simulink model "LoFT_Example3"  (R2024b)
settings: Solver=ode4  StartTime=0.0  StopTime=300  FixedStep=simu.dt  RelTol=1e-3
undefined symbols (not defined in the file): body, circtime, Communication, D1, Delta, irkb, line, LoFT, p0, Pn, s, simu, trip_time, Turbwind, waves, wind
libraries: simulink x350, spsThreePhaseVIMeasurementLib x41, spsThreePhasePISectionLineLib x34, spsThreePhaseParallelRLCLoadLib x21, spsThreePhaseTransformerTwoWindingsLib x14, spsLoadFlowBusLib x10, spsThreePhaseDynamicLoadLib x9, spsSynchronousMachinepuStandardLib x7, spsExcitationSystemLib x7, spsSteamTurbineandGovernorLib x7, spsGenericPowerSystemStabilizerLib x7, spsMultiBandPowerSystemStabilizerLib x7
(part 40 of 49)

== system LoFT_Example3/FOWT System/Subsystem11/FOWT6/Aerodynamics and Local Control Systems/Local Control Systems/Subsystem1 ==
  RotSpeed : Inport
  WindSpeed : Inport  Port=2
  3 : Inport  Port=3
  Nacelle Speed : Inport  Port=4
  1-D Lookup Table : Lookup_n-D  NumberOfTableDimensions=1  BreakpointsForDimension1=Controller.R.PS_WindSpeeds  Table=Controller.R.PS_BldPitchMin  InternalRulePriority=Speed  RndMeth=Simplest
  Compare To Constant : simulink/Logic and Bit Operations/Compare To Constant  relop=<=  const=0  OutDataTypeStr=boolean
  Constant : Constant  Value=7.55*pi/30
  Constant1 : Constant  Value=90*pi/180
  Delay : Delay  DelayLength=1  InitialCondition=0
  Divide3 : Product  Inputs=**
  Gain : Gain  Gain=Controller.KV *0.5
  Gain Scheduling : Subsystem
  Gain1 : Gain
  Rate Limiter : RateLimiter  RisingSlewLimit=2*pi/180  FallingSlewLimit=-2 * pi/180  SampleTimeMode=inherited
  Saturation : Saturate  UpperLimit=7.55*pi/30  LowerLimit=5*pi/30
  Saturation Dynamic : simulink/Discontinuities/Saturation Dynamic  OutMin=[]  OutMax=[]  OutDataTypeStr=Inherit: Same as second input  OutDataType=fixdt(1, 16)  OutScaling=2^-10  DoSatur=off
  Scope2 : Scope
  Sum1 : Sum  Inputs=|++
  Sum3 : Sum  Inputs=|+-
  Sum4 : Sum  Inputs=|+-
  BldPitch : Outport
  wires:
  Divide3/1 -> Sum4/2
  Sum3/1 -> Gain Scheduling/1(In1)
  Saturation Dynamic/1 -> Rate Limiter/1, Delay/1
  Compare To Constant/1 -> Divide3/1
  Constant/1 -> Sum4/1
  Constant1/1 -> Saturation Dynamic/1
  3/1 -> Compare To Constant/1, Divide3/2
  Delay/1 -> Gain Scheduling/3(In2)
  RotSpeed/1 -> Sum3/2
  Gain Scheduling/1(Out1) -> Sum1/1
  Sum1/1 -> Saturation Dynamic/2
  Gain/1 -> Sum1/2
  Nacelle Speed/1 -> Gain/1
  WindSpeed/1 -> 1-D Lookup Table/1  "Vhat"
  1-D Lookup Table/1 -> Gain1/1
  Gain1/1 -> Saturation Dynamic/3, Gain Scheduling/2(In3), Scope2/1
  Rate Limiter/1 -> BldPitch/1
  Sum4/1 -> Saturation/1
  Saturation/1 -> Sum3/1

== system LoFT_Example3/FOWT System/Subsystem11/FOWT6/Aerodynamics and Local Control Systems/Local Control Systems/Subsystem2 ==
  GenTorq : Inport
  BldPitch : Inport  Port=2
  Constant3 : Constant  Value=-Controller.torqueMax
  Gain 1 : Gain  Gain=Controller.SPS_kb/deg2rad(30)
  Gain 2 : Gain  Gain=Controller.omegaMax
  Gain 3 : Gain  Gain=-Controller.SPS_kt/Controller.torqueMax
  Sum5 : Sum  Inputs=|+-
  Sum6 : Sum  Inputs=|+-
  Delta_omega_g : Outport
  wires:
  Sum6/1 -> Gain 2/1
  Gain 1/1 -> Sum6/1
  Constant3/1 -> Sum5/2
  Gain 3/1 -> Sum6/2
  Sum5/1 -> Gain 3/1
  Gain 2/1 -> Delta_omega_g/1
  BldPitch/1 -> Gain 1/1
  GenTorq/1 -> Sum5/1

== system LoFT_Example3/FOWT System/Subsystem11/FOWT6/Aerodynamics and Local Control Systems/Local Control Systems/wind speed estimator ==
  In1 : Inport
  Discrete Filter : DiscreteFilter  Numerator=Controller.F.Wind.b  Denominator=Controller.F.Wind.a  InitialStates=2000
  Out1 : Outport
  wires:
  Discrete Filter/1 -> Out1/1
  In1/1 -> Discrete Filter/1

== system LoFT_Example3/FOWT System/Subsystem11/FOWT7/Aerodynamics and Local Control Systems/Local Control Systems/Subsystem ==
  WindSpeed : Inport
  2 : Inport  Port=2
  RotSpeed : Inport  Port=3
  Compare To Constant1 : simulink/Logic and Bit Operations/Compare To Constant  relop=>=  const=0  OutDataTypeStr=boolean
  Divide4 : Product  Inputs=**
  Gain5 : Gain  Gain=Controller.R.VS_KI
  Gain6 : Gain  Gain=Controller.R.VS_KP
  Integrator1 : Integrator  InitialCondition=Controller.torqueMax * 0.7  LimitOutput=on  UpperSaturationLimit=Controller.torqueMax
  Optimall TSR / Radius : Gain  Gain=Controller.R.VS_TSRopt/Controller.R.RotorRad
  Rate Limiter : RateLimiter  RisingSlewLimit=Controller.torqueMaxRate  FallingSlewLimit=-Controller.torqueMaxRate  SampleTimeMode=inherited
  Saturation : Saturate  UpperLimit=7.55*pi/30  LowerLimit=5*pi/30
  Saturation1 : Saturate  UpperLimit=Controller.torqueMax  LowerLimit=0
  Saturation2 : Saturate  UpperLimit=7.55*pi/30  LowerLimit=5*pi/30
  Scope2 : Scope
  Sum2 : Sum  Inputs=|+-
  Sum7 : Sum  Inputs=|+-
  Sum8 : Sum  Inputs=|++
  GenTorq : Outport
  wires:
  Gain6/1 -> Sum8/1
  WindSpeed/1 -> Optimall TSR / Radius/1
  Sum7/1 -> Saturation/1
  Divide4/1 -> Scope2/1, Sum7/2
  2/1 -> Compare To Constant1/1, Divide4/2
  Rate Limiter/1 -> GenTorq/1
  Saturation/1 -> Sum2/1
  Compare To Constant1/1 -> Divide4/1
  Sum2/1 -> Gain6/1, Gain5/1
  Integrator1/1 -> Sum8/2
  Gain5/1 -> Integrator1/1
  Sum8/1 -> Saturation1/1
  RotSpeed/1 -> Sum2/2
  Saturation1/1 -> Rate Limiter/1
  Saturation2/1 -> Sum7/1
  Optimall TSR / Radius/1 -> Saturation2/1

== system LoFT_Example3/FOWT System/Subsystem11/FOWT7/Aerodynamics and Local Control Systems/Local Control Systems/Subsystem1 ==
  RotSpeed : Inport
  WindSpeed : Inport  Port=2
  3 : Inport  Port=3
  Nacelle Speed : Inport  Port=4
  1-D Lookup Table : Lookup_n-D  NumberOfTableDimensions=1  BreakpointsForDimension1=Controller.R.PS_WindSpeeds  Table=Controller.R.PS_BldPitchMin  InternalRulePriority=Speed  RndMeth=Simplest
  Compare To Constant : simulink/Logic and Bit Operations/Compare To Constant  relop=<=  const=0  OutDataTypeStr=boolean
  Constant : Constant  Value=7.55*pi/30
  Constant1 : Constant  Value=90*pi/180
  Delay : Delay  DelayLength=1  InitialCondition=0
  Divide3 : Product  Inputs=**
  Gain : Gain  Gain=Controller.KV *0.5
  Gain Scheduling : Subsystem
  Gain1 : Gain
  Rate Limiter : RateLimiter  RisingSlewLimit=2*pi/180  FallingSlewLimit=-2 * pi/180  SampleTimeMode=inherited
  Saturation : Saturate  UpperLimit=7.55*pi/30  LowerLimit=5*pi/30
  Saturation Dynamic : simulink/Discontinuities/Saturation Dynamic  OutMin=[]  OutMax=[]  OutDataTypeStr=Inherit: Same as second input  OutDataType=fixdt(1, 16)  OutScaling=2^-10  DoSatur=off
  Scope2 : Scope
  Sum1 : Sum  Inputs=|++
  Sum3 : Sum  Inputs=|+-
  Sum4 : Sum  Inputs=|+-
  BldPitch : Outport
  wires:
  Saturation/1 -> Sum3/1
  Sum4/1 -> Saturation/1
  Rate Limiter/1 -> BldPitch/1
  Gain1/1 -> Scope2/1, Gain Scheduling/2(In3), Saturation Dynamic/3
  1-D Lookup Table/1 -> Gain1/1
  WindSpeed/1 -> 1-D Lookup Table/1  "Vhat"
  Nacelle Speed/1 -> Gain/1
  Gain/1 -> Sum1/2
  Sum1/1 -> Saturation Dynamic/2
  Gain Scheduling/1(Out1) -> Sum1/1
  RotSpeed/1 -> Sum3/2
  Delay/1 -> Gain Scheduling/3(In2)
  3/1 -> Divide3/2, Compare To Constant/1
  Constant1/1 -> Saturation Dynamic/1
  Constant/1 -> Sum4/1
  Compare To Constant/1 -> Divide3/1
  Saturation Dynamic/1 -> Delay/1, Rate Limiter/1
  Sum3/1 -> Gain Scheduling/1(In1)
  Divide3/1 -> Sum4/2

== system LoFT_Example3/FOWT System/Subsystem11/FOWT7/Aerodynamics and Local Control Systems/Local Control Systems/Subsystem2 ==
  GenTorq : Inport
  BldPitch : Inport  Port=2
  Constant3 : Constant  Value=-Controller.torqueMax
  Gain 1 : Gain  Gain=Controller.SPS_kb/deg2rad(30)
  Gain 2 : Gain  Gain=Controller.omegaMax
  Gain 3 : Gain  Gain=-Controller.SPS_kt/Controller.torqueMax
  Sum5 : Sum  Inputs=|+-
  Sum6 : Sum  Inputs=|+-
  Delta_omega_g : Outport
  wires:
  GenTorq/1 -> Sum5/1
  BldPitch/1 -> Gain 1/1
  Gain 2/1 -> Delta_omega_g/1
  Sum5/1 -> Gain 3/1
  Gain 3/1 -> Sum6/2
  Constant3/1 -> Sum5/2
  Gain 1/1 -> Sum6/1
  Sum6/1 -> Gain 2/1

== system LoFT_Example3/FOWT System/Subsystem11/FOWT7/Aerodynamics and Local Control Systems/Local Control Systems/wind speed estimator ==
  In1 : Inport
  Discrete Filter : DiscreteFilter  Numerator=Controller.F.Wind.b  Denominator=Controller.F.Wind.a  InitialStates=2000
  Out1 : Outport
  wires:
  In1/1 -> Discrete Filter/1
  Discrete Filter/1 -> Out1/1

== system LoFT_Example3/FOWT System/Subsystem11/FOWT8/Aerodynamics and Local Control Systems/Local Control Systems/Subsystem ==
  WindSpeed : Inport
  2 : Inport  Port=2
  RotSpeed : Inport  Port=3
  Compare To Constant1 : simulink/Logic and Bit Operations/Compare To Constant  relop=>=  const=0  OutDataTypeStr=boolean
  Divide4 : Product  Inputs=**
  Gain5 : Gain  Gain=Controller.R.VS_KI
  Gain6 : Gain  Gain=Controller.R.VS_KP
  Integrator1 : Integrator  InitialCondition=Controller.torqueMax * 0.7  LimitOutput=on  UpperSaturationLimit=Controller.torqueMax
  Optimall TSR / Radius : Gain  Gain=Controller.R.VS_TSRopt/Controller.R.RotorRad
  Rate Limiter : RateLimiter  RisingSlewLimit=Controller.torqueMaxRate  FallingSlewLimit=-Controller.torqueMaxRate  SampleTimeMode=inherited
  Saturation : Saturate  UpperLimit=7.55*pi/30  LowerLimit=5*pi/30
  Saturation1 : Saturate  UpperLimit=Controller.torqueMax  LowerLimit=0
  Saturation2 : Saturate  UpperLimit=7.55*pi/30  LowerLimit=5*pi/30
  Scope2 : Scope
  Sum2 : Sum  Inputs=|+-
  Sum7 : Sum  Inputs=|+-
  Sum8 : Sum  Inputs=|++
  GenTorq : Outport
  wires:
  Optimall TSR / Radius/1 -> Saturation2/1
  Saturation2/1 -> Sum7/1
  Saturation1/1 -> Rate Limiter/1
  RotSpeed/1 -> Sum2/2
  Sum8/1 -> Saturation1/1
  Gain5/1 -> Integrator1/1
  Integrator1/1 -> Sum8/2
  Sum2/1 -> Gain5/1, Gain6/1
  Compare To Constant1/1 -> Divide4/1
  Saturation/1 -> Sum2/1
  Rate Limiter/1 -> GenTorq/1
  2/1 -> Divide4/2, Compare To Constant1/1
  Divide4/1 -> Sum7/2, Scope2/1
  Sum7/1 -> Saturation/1
  WindSpeed/1 -> Optimall TSR / Radius/1
  Gain6/1 -> Sum8/1

== system LoFT_Example3/FOWT System/Subsystem11/FOWT8/Aerodynamics and Local Control Systems/Local Control Systems/Subsystem1 ==
  RotSpeed : Inport
  WindSpeed : Inport  Port=2
  3 : Inport  Port=3
  Nacelle Speed : Inport  Port=4
  1-D Lookup Table : Lookup_n-D  NumberOfTableDimensions=1  BreakpointsForDimension1=Controller.R.PS_WindSpeeds  Table=Controller.R.PS_BldPitchMin  InternalRulePriority=Speed  RndMeth=Simplest
  Compare To Constant : simulink/Logic and Bit Operations/Compare To Constant  relop=<=  const=0  OutDataTypeStr=boolean
  Constant : Constant  Value=7.55*pi/30
  Constant1 : Constant  Value=90*pi/180
  Delay : Delay  DelayLength=1  InitialCondition=0
  Divide3 : Product  Inputs=**
  Gain : Gain  Gain=Controller.KV *0.5
  Gain Scheduling : Subsystem
  Gain1 : Gain
  Rate Limiter : RateLimiter  RisingSlewLimit=2*pi/180  FallingSlewLimit=-2 * pi/180  SampleTimeMode=inherited
  Saturation : Saturate  UpperLimit=7.55*pi/30  LowerLimit=5*pi/30
  Saturation Dynamic : simulink/Discontinuities/Saturation Dynamic  OutMin=[]  OutMax=[]  OutDataTypeStr=Inherit: Same as second input  OutDataType=fixdt(1, 16)  OutScaling=2^-10  DoSatur=off
  Scope2 : Scope
  Sum1 : Sum  Inputs=|++
  Sum3 : Sum  Inputs=|+-
  Sum4 : Sum  Inputs=|+-
  BldPitch : Outport
  wires:
  Divide3/1 -> Sum4/2
  Sum3/1 -> Gain Scheduling/1(In1)
  Saturation Dynamic/1 -> Rate Limiter/1, Delay/1
  Compare To Constant/1 -> Divide3/1
  Constant/1 -> Sum4/1
  Constant1/1 -> Saturation Dynamic/1
  3/1 -> Compare To Constant/1, Divide3/2
  Delay/1 -> Gain Scheduling/3(In2)
  RotSpeed/1 -> Sum3/2
  Gain Scheduling/1(Out1) -> Sum1/1
  Sum1/1 -> Saturation Dynamic/2
  Gain/1 -> Sum1/2
  Nacelle Speed/1 -> Gain/1
  WindSpeed/1 -> 1-D Lookup Table/1  "Vhat"
  1-D Lookup Table/1 -> Gain1/1
  Gain1/1 -> Saturation Dynamic/3, Gain Scheduling/2(In3), Scope2/1
  Rate Limiter/1 -> BldPitch/1
  Sum4/1 -> Saturation/1
  Saturation/1 -> Sum3/1

== system LoFT_Example3/FOWT System/Subsystem11/FOWT8/Aerodynamics and Local Control Systems/Local Control Systems/Subsystem2 ==
  GenTorq : Inport
  BldPitch : Inport  Port=2
  Constant3 : Constant  Value=-Controller.torqueMax
  Gain 1 : Gain  Gain=Controller.SPS_kb/deg2rad(30)
  Gain 2 : Gain  Gain=Controller.omegaMax
  Gain 3 : Gain  Gain=-Controller.SPS_kt/Controller.torqueMax
  Sum5 : Sum  Inputs=|+-
  Sum6 : Sum  Inputs=|+-
  Delta_omega_g : Outport
  wires:
  Sum6/1 -> Gain 2/1
  Gain 1/1 -> Sum6/1
  Constant3/1 -> Sum5/2
  Gain 3/1 -> Sum6/2
  Sum5/1 -> Gain 3/1
  Gain 2/1 -> Delta_omega_g/1
  BldPitch/1 -> Gain 1/1
  GenTorq/1 -> Sum5/1

== system LoFT_Example3/FOWT System/Subsystem11/FOWT8/Aerodynamics and Local Control Systems/Local Control Systems/wind speed estimator ==
  In1 : Inport
  Discrete Filter : DiscreteFilter  Numerator=Controller.F.Wind.b  Denominator=Controller.F.Wind.a  InitialStates=2000
  Out1 : Outport
  wires:
  Discrete Filter/1 -> Out1/1
  In1/1 -> Discrete Filter/1

== system LoFT_Example3/FOWT System/Subsystem11/FOWT9/Aerodynamics and Local Control Systems/Local Control Systems/Subsystem ==
  WindSpeed : Inport
  2 : Inport  Port=2
  RotSpeed : Inport  Port=3
  Compare To Constant1 : simulink/Logic and Bit Operations/Compare To Constant  relop=>=  const=0  OutDataTypeStr=boolean
  Divide4 : Product  Inputs=**
  Gain5 : Gain  Gain=Controller.R.VS_KI
  Gain6 : Gain  Gain=Controller.R.VS_KP
  Integrator1 : Integrator  InitialCondition=Controller.torqueMax * 0.7  LimitOutput=on  UpperSaturationLimit=Controller.torqueMax
  Optimall TSR / Radius : Gain  Gain=Controller.R.VS_TSRopt/Controller.R.RotorRad
  Rate Limiter : RateLimiter  RisingSlewLimit=Controller.torqueMaxRate  FallingSlewLimit=-Controller.torqueMaxRate  SampleTimeMode=inherited
  Saturation : Saturate  UpperLimit=7.55*pi/30  LowerLimit=5*pi/30
  Saturation1 : Saturate  UpperLimit=Controller.torqueMax  LowerLimit=0
  Saturation2 : Saturate  UpperLimit=7.55*pi/30  LowerLimit=5*pi/30
  Scope2 : Scope
  Sum2 : Sum  Inputs=|+-
  Sum7 : Sum  Inputs=|+-
  Sum8 : Sum  Inputs=|++
  GenTorq : Outport
  wires:
  Gain6/1 -> Sum8/1
  WindSpeed/1 -> Optimall TSR / Radius/1
  Sum7/1 -> Saturation/1
  Divide4/1 -> Scope2/1, Sum7/2
  2/1 -> Compare To Constant1/1, Divide4/2
  Rate Limiter/1 -> GenTorq/1
  Saturation/1 -> Sum2/1
  Compare To Constant1/1 -> Divide4/1
  Sum2/1 -> Gain6/1, Gain5/1
  Integrator1/1 -> Sum8/2
  Gain5/1 -> Integrator1/1
  Sum8/1 -> Saturation1/1
  RotSpeed/1 -> Sum2/2
  Saturation1/1 -> Rate Limiter/1
  Saturation2/1 -> Sum7/1
  Optimall TSR / Radius/1 -> Saturation2/1

== system LoFT_Example3/FOWT System/Subsystem11/FOWT9/Aerodynamics and Local Control Systems/Local Control Systems/Subsystem1 ==
  RotSpeed : Inport
  WindSpeed : Inport  Port=2
  3 : Inport  Port=3
  Nacelle Speed : Inport  Port=4
  1-D Lookup Table : Lookup_n-D  NumberOfTableDimensions=1  BreakpointsForDimension1=Controller.R.PS_WindSpeeds  Table=Controller.R.PS_BldPitchMin  InternalRulePriority=Speed  RndMeth=Simplest
  Compare To Constant : simulink/Logic and Bit Operations/Compare To Constant  relop=<=  const=0  OutDataTypeStr=boolean
  Constant : Constant  Value=7.55*pi/30
  Constant1 : Constant  Value=90*pi/180
  Delay : Delay  DelayLength=1  InitialCondition=0
  Divide3 : Product  Inputs=**
  Gain : Gain  Gain=Controller.KV *0.5
  Gain Scheduling : Subsystem
  Gain1 : Gain
  Rate Limiter : RateLimiter  RisingSlewLimit=2*pi/180  FallingSlewLimit=-2 * pi/180  SampleTimeMode=inherited
  Saturation : Saturate  UpperLimit=7.55*pi/30  LowerLimit=5*pi/30
  Saturation Dynamic : simulink/Discontinuities/Saturation Dynamic  OutMin=[]  OutMax=[]  OutDataTypeStr=Inherit: Same as second input  OutDataType=fixdt(1, 16)  OutScaling=2^-10  DoSatur=off
  Scope2 : Scope
  Sum1 : Sum  Inputs=|++
  Sum3 : Sum  Inputs=|+-
  Sum4 : Sum  Inputs=|+-
  BldPitch : Outport
  wires:
  Saturation/1 -> Sum3/1
  Sum4/1 -> Saturation/1
  Rate Limiter/1 -> BldPitch/1
  Gain1/1 -> Scope2/1, Gain Scheduling/2(In3), Saturation Dynamic/3
  1-D Lookup Table/1 -> Gain1/1
  WindSpeed/1 -> 1-D Lookup Table/1  "Vhat"
  Nacelle Speed/1 -> Gain/1
  Gain/1 -> Sum1/2
  Sum1/1 -> Saturation Dynamic/2
  Gain Scheduling/1(Out1) -> Sum1/1
  RotSpeed/1 -> Sum3/2
  Delay/1 -> Gain Scheduling/3(In2)
  3/1 -> Divide3/2, Compare To Constant/1
  Constant1/1 -> Saturation Dynamic/1
  Constant/1 -> Sum4/1
  Compare To Constant/1 -> Divide3/1
  Saturation Dynamic/1 -> Delay/1, Rate Limiter/1
  Sum3/1 -> Gain Scheduling/1(In1)
  Divide3/1 -> Sum4/2

== system LoFT_Example3/FOWT System/Subsystem11/FOWT9/Aerodynamics and Local Control Systems/Local Control Systems/Subsystem2 ==
  GenTorq : Inport
  BldPitch : Inport  Port=2
  Constant3 : Constant  Value=-Controller.torqueMax
  Gain 1 : Gain  Gain=Controller.SPS_kb/deg2rad(30)
  Gain 2 : Gain  Gain=Controller.omegaMax
  Gain 3 : Gain  Gain=-Controller.SPS_kt/Controller.torqueMax
  Sum5 : Sum  Inputs=|+-
  Sum6 : Sum  Inputs=|+-
  Delta_omega_g : Outport
  wires:
  GenTorq/1 -> Sum5/1
  BldPitch/1 -> Gain 1/1
  Gain 2/1 -> Delta_omega_g/1
  Sum5/1 -> Gain 3/1
  Gain 3/1 -> Sum6/2
  Constant3/1 -> Sum5/2
  Gain 1/1 -> Sum6/1
  Sum6/1 -> Gain 2/1

== system LoFT_Example3/FOWT System/Subsystem11/FOWT9/Aerodynamics and Local Control Systems/Local Control Systems/wind speed estimator ==
  In1 : Inport
  Discrete Filter : DiscreteFilter  Numerator=Controller.F.Wind.b  Denominator=Controller.F.Wind.a  InitialStates=2000
  Out1 : Outport
  wires:
  In1/1 -> Discrete Filter/1
  Discrete Filter/1 -> Out1/1

== system LoFT_Example3/FOWT System/Subsystem13/FOWT1/Aerodynamics and Local Control Systems/Local Control Systems/Subsystem ==
  WindSpeed : Inport
  2 : Inport  Port=2
  RotSpeed : Inport  Port=3
  Compare To Constant1 : simulink/Logic and Bit Operations/Compare To Constant  relop=>=  const=0  OutDataTypeStr=boolean
  Divide4 : Product  Inputs=**
  Gain5 : Gain  Gain=Controller.R.VS_KI
  Gain6 : Gain  Gain=Controller.R.VS_KP
  Integrator1 : Integrator  InitialCondition=Controller.torqueMax * 0.7  LimitOutput=on  UpperSaturationLimit=Controller.torqueMax
  Optimall TSR / Radius : Gain  Gain=Controller.R.VS_TSRopt/Controller.R.RotorRad
  Rate Limiter : RateLimiter  RisingSlewLimit=Controller.torqueMaxRate  FallingSlewLimit=-Controller.torqueMaxRate  SampleTimeMode=inherited
  Saturation : Saturate  UpperLimit=7.55*pi/30  LowerLimit=5*pi/30
  Saturation1 : Saturate  UpperLimit=Controller.torqueMax  LowerLimit=0
  Saturation2 : Saturate  UpperLimit=7.55*pi/30  LowerLimit=5*pi/30
  Scope2 : Scope
  Sum2 : Sum  Inputs=|+-
  Sum7 : Sum  Inputs=|+-
  Sum8 : Sum  Inputs=|++
  GenTorq : Outport
  wires:
  Optimall TSR / Radius/1 -> Saturation2/1
  Saturation2/1 -> Sum7/1
  Saturation1/1 -> Rate Limiter/1
  RotSpeed/1 -> Sum2/2
  Sum8/1 -> Saturation1/1
  Gain5/1 -> Integrator1/1
  Integrator1/1 -> Sum8/2
  Sum2/1 -> Gain5/1, Gain6/1
  Compare To Constant1/1 -> Divide4/1
  Saturation/1 -> Sum2/1
  Rate Limiter/1 -> GenTorq/1
  2/1 -> Divide4/2, Compare To Constant1/1
  Divide4/1 -> Sum7/2, Scope2/1
  Sum7/1 -> Saturation/1
  WindSpeed/1 -> Optimall TSR / Radius/1
  Gain6/1 -> Sum8/1

== system LoFT_Example3/FOWT System/Subsystem13/FOWT1/Aerodynamics and Local Control Systems/Local Control Systems/Subsystem1 ==
  RotSpeed : Inport
  WindSpeed : Inport  Port=2
  3 : Inport  Port=3
  Nacelle Speed : Inport  Port=4
  1-D Lookup Table : Lookup_n-D  NumberOfTableDimensions=1  BreakpointsForDimension1=Controller.R.PS_WindSpeeds  Table=Controller.R.PS_BldPitchMin  InternalRulePriority=Speed  RndMeth=Simplest
  Compare To Constant : simulink/Logic and Bit Operations/Compare To Constant  relop=<=  const=0  OutDataTypeStr=boolean
  Constant : Constant  Value=7.55*pi/30
  Constant1 : Constant  Value=90*pi/180
  Delay : Delay  DelayLength=1  InitialCondition=0
  Divide3 : Product  Inputs=**
  Gain : Gain  Gain=Controller.KV *0.5
  Gain Scheduling : Subsystem
  Gain1 : Gain
  Rate Limiter : RateLimiter  RisingSlewLimit=2*pi/180  FallingSlewLimit=-2 * pi/180  SampleTimeMode=inherited
  Saturation : Saturate  UpperLimit=7.55*pi/30  LowerLimit=5*pi/30
  Saturation Dynamic : simulink/Discontinuities/Saturation Dynamic  OutMin=[]  OutMax=[]  OutDataTypeStr=Inherit: Same as second input  OutDataType=fixdt(1, 16)  OutScaling=2^-10  DoSatur=off
  Scope2 : Scope
  Sum1 : Sum  Inputs=|++
  Sum3 : Sum  Inputs=|+-
  Sum4 : Sum  Inputs=|+-
  BldPitch : Outport
  wires:
  Divide3/1 -> Sum4/2
  Sum3/1 -> Gain Scheduling/1(In1)
  Saturation Dynamic/1 -> Rate Limiter/1, Delay/1
  Compare To Constant/1 -> Divide3/1
  Constant/1 -> Sum4/1
  Constant1/1 -> Saturation Dynamic/1
  3/1 -> Compare To Constant/1, Divide3/2
  Delay/1 -> Gain Scheduling/3(In2)
  RotSpeed/1 -> Sum3/2
  Gain Scheduling/1(Out1) -> Sum1/1
  Sum1/1 -> Saturation Dynamic/2
  Gain/1 -> Sum1/2
  Nacelle Speed/1 -> Gain/1
  WindSpeed/1 -> 1-D Lookup Table/1  "Vhat"
  1-D Lookup Table/1 -> Gain1/1
  Gain1/1 -> Saturation Dynamic/3, Gain Scheduling/2(In3), Scope2/1
  Rate Limiter/1 -> BldPitch/1
  Sum4/1 -> Saturation/1
  Saturation/1 -> Sum3/1

== system LoFT_Example3/FOWT System/Subsystem13/FOWT1/Aerodynamics and Local Control Systems/Local Control Systems/Subsystem2 ==
  GenTorq : Inport
  BldPitch : Inport  Port=2
  Constant3 : Constant  Value=-Controller.torqueMax
  Gain 1 : Gain  Gain=Controller.SPS_kb/deg2rad(30)
  Gain 2 : Gain  Gain=Controller.omegaMax
  Gain 3 : Gain  Gain=-Controller.SPS_kt/Controller.torqueMax
  Sum5 : Sum  Inputs=|+-
  Sum6 : Sum  Inputs=|+-
  Delta_omega_g : Outport
  wires:
  Sum6/1 -> Gain 2/1
  Gain 1/1 -> Sum6/1
  Constant3/1 -> Sum5/2
  Gain 3/1 -> Sum6/2
  Sum5/1 -> Gain 3/1
  Gain 2/1 -> Delta_omega_g/1
  BldPitch/1 -> Gain 1/1
  GenTorq/1 -> Sum5/1

== system LoFT_Example3/FOWT System/Subsystem13/FOWT1/Aerodynamics and Local Control Systems/Local Control Systems/wind speed estimator ==
  In1 : Inport
  Discrete Filter : DiscreteFilter  Numerator=Controller.F.Wind.b  Denominator=Controller.F.Wind.a  InitialStates=2000
  Out1 : Outport
  wires:
  Discrete Filter/1 -> Out1/1
  In1/1 -> Discrete Filter/1

== system LoFT_Example3/FOWT System/Subsystem13/FOWT10/Aerodynamics and Local Control Systems/Local Control Systems/Subsystem ==
  WindSpeed : Inport
  2 : Inport  Port=2
  RotSpeed : Inport  Port=3
  Compare To Constant1 : simulink/Logic and Bit Operations/Compare To Constant  relop=>=  const=0  OutDataTypeStr=boolean
  Divide4 : Product  Inputs=**
  Gain5 : Gain  Gain=Controller.R.VS_KI
  Gain6 : Gain  Gain=Controller.R.VS_KP
  Integrator1 : Integrator  InitialCondition=Controller.torqueMax * 0.7  LimitOutput=on  UpperSaturationLimit=Controller.torqueMax
  Optimall TSR / Radius : Gain  Gain=Controller.R.VS_TSRopt/Controller.R.RotorRad
  Rate Limiter : RateLimiter  RisingSlewLimit=Controller.torqueMaxRate  FallingSlewLimit=-Controller.torqueMaxRate  SampleTimeMode=inherited
  Saturation : Saturate  UpperLimit=7.55*pi/30  LowerLimit=5*pi/30
  Saturation1 : Saturate  UpperLimit=Controller.torqueMax  LowerLimit=0
  Saturation2 : Saturate  UpperLimit=7.55*pi/30  LowerLimit=5*pi/30
  Scope2 : Scope
  Sum2 : Sum  Inputs=|+-
  Sum7 : Sum  Inputs=|+-
  Sum8 : Sum  Inputs=|++
  GenTorq : Outport
  wires:
  Gain6/1 -> Sum8/1
  WindSpeed/1 -> Optimall TSR / Radius/1
  Sum7/1 -> Saturation/1
  Divide4/1 -> Scope2/1, Sum7/2
  2/1 -> Compare To Constant1/1, Divide4/2
  Rate Limiter/1 -> GenTorq/1
  Saturation/1 -> Sum2/1
  Compare To Constant1/1 -> Divide4/1
  Sum2/1 -> Gain6/1, Gain5/1
  Integrator1/1 -> Sum8/2
  Gain5/1 -> Integrator1/1
  Sum8/1 -> Saturation1/1
  RotSpeed/1 -> Sum2/2
  Saturation1/1 -> Rate Limiter/1
  Saturation2/1 -> Sum7/1
  Optimall TSR / Radius/1 -> Saturation2/1

== system LoFT_Example3/FOWT System/Subsystem13/FOWT10/Aerodynamics and Local Control Systems/Local Control Systems/Subsystem1 ==
  RotSpeed : Inport
  WindSpeed : Inport  Port=2
  3 : Inport  Port=3
  Nacelle Speed : Inport  Port=4
  1-D Lookup Table : Lookup_n-D  NumberOfTableDimensions=1  BreakpointsForDimension1=Controller.R.PS_WindSpeeds  Table=Controller.R.PS_BldPitchMin  InternalRulePriority=Speed  RndMeth=Simplest
  Compare To Constant : simulink/Logic and Bit Operations/Compare To Constant  relop=<=  const=0  OutDataTypeStr=boolean
  Constant : Constant  Value=7.55*pi/30
  Constant1 : Constant  Value=90*pi/180
  Delay : Delay  DelayLength=1  InitialCondition=0
  Divide3 : Product  Inputs=**
  Gain : Gain  Gain=Controller.KV *0.5
  Gain Scheduling : Subsystem
  Gain1 : Gain
  Rate Limiter : RateLimiter  RisingSlewLimit=2*pi/180  FallingSlewLimit=-2 * pi/180  SampleTimeMode=inherited
  Saturation : Saturate  UpperLimit=7.55*pi/30  LowerLimit=5*pi/30
  Saturation Dynamic : simulink/Discontinuities/Saturation Dynamic  OutMin=[]  OutMax=[]  OutDataTypeStr=Inherit: Same as second input  OutDataType=fixdt(1, 16)  OutScaling=2^-10  DoSatur=off
  Scope2 : Scope
  Sum1 : Sum  Inputs=|++
  Sum3 : Sum  Inputs=|+-
  Sum4 : Sum  Inputs=|+-
  BldPitch : Outport
  wires:
  Saturation/1 -> Sum3/1
  Sum4/1 -> Saturation/1
  Rate Limiter/1 -> BldPitch/1
  Gain1/1 -> Scope2/1, Gain Scheduling/2(In3), Saturation Dynamic/3
  1-D Lookup Table/1 -> Gain1/1
  WindSpeed/1 -> 1-D Lookup Table/1  "Vhat"
  Nacelle Speed/1 -> Gain/1
  Gain/1 -> Sum1/2
  Sum1/1 -> Saturation Dynamic/2
  Gain Scheduling/1(Out1) -> Sum1/1
  RotSpeed/1 -> Sum3/2
  Delay/1 -> Gain Scheduling/3(In2)
  3/1 -> Divide3/2, Compare To Constant/1
  Constant1/1 -> Saturation Dynamic/1
  Constant/1 -> Sum4/1
  Compare To Constant/1 -> Divide3/1
  Saturation Dynamic/1 -> Delay/1, Rate Limiter/1
  Sum3/1 -> Gain Scheduling/1(In1)
  Divide3/1 -> Sum4/2

== system LoFT_Example3/FOWT System/Subsystem13/FOWT10/Aerodynamics and Local Control Systems/Local Control Systems/Subsystem2 ==
  GenTorq : Inport
  BldPitch : Inport  Port=2
  Constant3 : Constant  Value=-Controller.torqueMax
  Gain 1 : Gain  Gain=Controller.SPS_kb/deg2rad(30)
  Gain 2 : Gain  Gain=Controller.omegaMax
  Gain 3 : Gain  Gain=-Controller.SPS_kt/Controller.torqueMax
  Sum5 : Sum  Inputs=|+-
  Sum6 : Sum  Inputs=|+-
  Delta_omega_g : Outport
  wires:
  GenTorq/1 -> Sum5/1
  BldPitch/1 -> Gain 1/1
  Gain 2/1 -> Delta_omega_g/1
  Sum5/1 -> Gain 3/1
  Gain 3/1 -> Sum6/2
  Constant3/1 -> Sum5/2
  Gain 1/1 -> Sum6/1
  Sum6/1 -> Gain 2/1

== system LoFT_Example3/FOWT System/Subsystem13/FOWT10/Aerodynamics and Local Control Systems/Local Control Systems/wind speed estimator ==
  In1 : Inport
  Discrete Filter : DiscreteFilter  Numerator=Controller.F.Wind.b  Denominator=Controller.F.Wind.a  InitialStates=2000
  Out1 : Outport
  wires:
  In1/1 -> Discrete Filter/1
  Discrete Filter/1 -> Out1/1

== system LoFT_Example3/FOWT System/Subsystem13/FOWT2/Aerodynamics and Local Control Systems/Local Control Systems/Subsystem ==
  WindSpeed : Inport
  2 : Inport  Port=2
  RotSpeed : Inport  Port=3
  Compare To Constant1 : simulink/Logic and Bit Operations/Compare To Constant  relop=>=  const=0  OutDataTypeStr=boolean
  Divide4 : Product  Inputs=**
  Gain5 : Gain  Gain=Controller.R.VS_KI
  Gain6 : Gain  Gain=Controller.R.VS_KP
  Integrator1 : Integrator  InitialCondition=Controller.torqueMax * 0.7  LimitOutput=on  UpperSaturationLimit=Controller.torqueMax
  Optimall TSR / Radius : Gain  Gain=Controller.R.VS_TSRopt/Controller.R.RotorRad
  Rate Limiter : RateLimiter  RisingSlewLimit=Controller.torqueMaxRate  FallingSlewLimit=-Controller.torqueMaxRate  SampleTimeMode=inherited
  Saturation : Saturate  UpperLimit=7.55*pi/30  LowerLimit=5*pi/30
  Saturation1 : Saturate  UpperLimit=Controller.torqueMax  LowerLimit=0
  Saturation2 : Saturate  UpperLimit=7.55*pi/30  LowerLimit=5*pi/30
  Scope2 : Scope
  Sum2 : Sum  Inputs=|+-
  Sum7 : Sum  Inputs=|+-
  Sum8 : Sum  Inputs=|++
  GenTorq : Outport
  wires:
  Gain6/1 -> Sum8/1
  WindSpeed/1 -> Optimall TSR / Radius/1
  Sum7/1 -> Saturation/1
  Divide4/1 -> Scope2/1, Sum7/2
  2/1 -> Compare To Constant1/1, Divide4/2
  Rate Limiter/1 -> GenTorq/1
  Saturation/1 -> Sum2/1
  Compare To Constant1/1 -> Divide4/1
  Sum2/1 -> Gain6/1, Gain5/1
  Integrator1/1 -> Sum8/2
  Gain5/1 -> Integrator1/1
  Sum8/1 -> Saturation1/1
  RotSpeed/1 -> Sum2/2
  Saturation1/1 -> Rate Limiter/1
  Saturation2/1 -> Sum7/1
  Optimall TSR / Radius/1 -> Saturation2/1

== system LoFT_Example3/FOWT System/Subsystem13/FOWT2/Aerodynamics and Local Control Systems/Local Control Systems/Subsystem1 ==
  RotSpeed : Inport
  WindSpeed : Inport  Port=2
  3 : Inport  Port=3
  Nacelle Speed : Inport  Port=4
  1-D Lookup Table : Lookup_n-D  NumberOfTableDimensions=1  BreakpointsForDimension1=Controller.R.PS_WindSpeeds  Table=Controller.R.PS_BldPitchMin  InternalRulePriority=Speed  RndMeth=Simplest
  Compare To Constant : simulink/Logic and Bit Operations/Compare To Constant  relop=<=  const=0  OutDataTypeStr=boolean
  Constant : Constant  Value=7.55*pi/30
  Constant1 : Constant  Value=90*pi/180
  Delay : Delay  DelayLength=1  InitialCondition=0
  Divide3 : Product  Inputs=**
  Gain : Gain  Gain=Controller.KV *0.5
  Gain Scheduling : Subsystem
  Gain1 : Gain
  Rate Limiter : RateLimiter  RisingSlewLimit=2*pi/180  FallingSlewLimit=-2 * pi/180  SampleTimeMode=inherited
  Saturation : Saturate  UpperLimit=7.55*pi/30  LowerLimit=5*pi/30
  Saturation Dynamic : simulink/Discontinuities/Saturation Dynamic  OutMin=[]  OutMax=[]  OutDataTypeStr=Inherit: Same as second input  OutDataType=fixdt(1, 16)  OutScaling=2^-10  DoSatur=off
  Scope2 : Scope
  Sum1 : Sum  Inputs=|++
  Sum3 : Sum  Inputs=|+-
  Sum4 : Sum  Inputs=|+-
  BldPitch : Outport
  wires:
  Saturation/1 -> Sum3/1
  Sum4/1 -> Saturation/1
  Rate Limiter/1 -> BldPitch/1
  Gain1/1 -> Scope2/1, Gain Scheduling/2(In3), Saturation Dynamic/3
  1-D Lookup Table/1 -> Gain1/1
  WindSpeed/1 -> 1-D Lookup Table/1  "Vhat"
  Nacelle Speed/1 -> Gain/1
  Gain/1 -> Sum1/2
  Sum1/1 -> Saturation Dynamic/2
  Gain Scheduling/1(Out1) -> Sum1/1
  RotSpeed/1 -> Sum3/2
  Delay/1 -> Gain Scheduling/3(In2)
  3/1 -> Divide3/2, Compare To Constant/1
  Constant1/1 -> Saturation Dynamic/1
  Constant/1 -> Sum4/1
  Compare To Constant/1 -> Divide3/1
  Saturation Dynamic/1 -> Delay/1, Rate Limiter/1
  Sum3/1 -> Gain Scheduling/1(In1)
  Divide3/1 -> Sum4/2

== system LoFT_Example3/FOWT System/Subsystem13/FOWT2/Aerodynamics and Local Control Systems/Local Control Systems/Subsystem2 ==
  GenTorq : Inport
  BldPitch : Inport  Port=2
  Constant3 : Constant  Value=-Controller.torqueMax
  Gain 1 : Gain  Gain=Controller.SPS_kb/deg2rad(30)
  Gain 2 : Gain  Gain=Controller.omegaMax
  Gain 3 : Gain  Gain=-Controller.SPS_kt/Controller.torqueMax
  Sum5 : Sum  Inputs=|+-
  Sum6 : Sum  Inputs=|+-
  Delta_omega_g : Outport
  wires:
  GenTorq/1 -> Sum5/1
  BldPitch/1 -> Gain 1/1
  Gain 2/1 -> Delta_omega_g/1
  Sum5/1 -> Gain 3/1
  Gain 3/1 -> Sum6/2
  Constant3/1 -> Sum5/2
  Gain 1/1 -> Sum6/1
  Sum6/1 -> Gain 2/1

== system LoFT_Example3/FOWT System/Subsystem13/FOWT2/Aerodynamics and Local Control Systems/Local Control Systems/wind speed estimator ==
  In1 : Inport
  Discrete Filter : DiscreteFilter  Numerator=Controller.F.Wind.b  Denominator=Controller.F.Wind.a  InitialStates=2000
  Out1 : Outport
  wires:
  In1/1 -> Discrete Filter/1
  Discrete Filter/1 -> Out1/1

== system LoFT_Example3/FOWT System/Subsystem13/FOWT3/Aerodynamics and Local Control Systems/Local Control Systems/Subsystem ==
  WindSpeed : Inport
  2 : Inport  Port=2
  RotSpeed : Inport  Port=3
  Compare To Constant1 : simulink/Logic and Bit Operations/Compare To Constant  relop=>=  const=0  OutDataTypeStr=boolean
  Divide4 : Product  Inputs=**
  Gain5 : Gain  Gain=Controller.R.VS_KI
  Gain6 : Gain  Gain=Controller.R.VS_KP
  Integrator1 : Integrator  InitialCondition=Controller.torqueMax * 0.7  LimitOutput=on  UpperSaturationLimit=Controller.torqueMax
  Optimall TSR / Radius : Gain  Gain=Controller.R.VS_TSRopt/Controller.R.RotorRad
  Rate Limiter : RateLimiter  RisingSlewLimit=Controller.torqueMaxRate  FallingSlewLimit=-Controller.torqueMaxRate  SampleTimeMode=inherited
  Saturation : Saturate  UpperLimit=7.55*pi/30  LowerLimit=5*pi/30
  Saturation1 : Saturate  UpperLimit=Controller.torqueMax  LowerLimit=0
  Saturation2 : Saturate  UpperLimit=7.55*pi/30  LowerLimit=5*pi/30
  Scope2 : Scope
  Sum2 : Sum  Inputs=|+-
  Sum7 : Sum  Inputs=|+-
  Sum8 : Sum  Inputs=|++
  GenTorq : Outport
  wires:
  Optimall TSR / Radius/1 -> Saturation2/1
  Saturation2/1 -> Sum7/1
  Saturation1/1 -> Rate Limiter/1
  RotSpeed/1 -> Sum2/2
  Sum8/1 -> Saturation1/1
  Gain5/1 -> Integrator1/1
  Integrator1/1 -> Sum8/2
  Sum2/1 -> Gain5/1, Gain6/1
  Compare To Constant1/1 -> Divide4/1
  Saturation/1 -> Sum2/1
  Rate Limiter/1 -> GenTorq/1
  2/1 -> Divide4/2, Compare To Constant1/1
  Divide4/1 -> Sum7/2, Scope2/1
  Sum7/1 -> Saturation/1
  WindSpeed/1 -> Optimall TSR / Radius/1
  Gain6/1 -> Sum8/1

== system LoFT_Example3/FOWT System/Subsystem13/FOWT3/Aerodynamics and Local Control Systems/Local Control Systems/Subsystem1 ==
  RotSpeed : Inport
  WindSpeed : Inport  Port=2
  3 : Inport  Port=3
  Nacelle Speed : Inport  Port=4
  1-D Lookup Table : Lookup_n-D  NumberOfTableDimensions=1  BreakpointsForDimension1=Controller.R.PS_WindSpeeds  Table=Controller.R.PS_BldPitchMin  InternalRulePriority=Speed  RndMeth=Simplest
  Compare To Constant : simulink/Logic and Bit Operations/Compare To Constant  relop=<=  const=0  OutDataTypeStr=boolean
  Constant : Constant  Value=7.55*pi/30
  Constant1 : Constant  Value=90*pi/180
  Delay : Delay  DelayLength=1  InitialCondition=0
  Divide3 : Product  Inputs=**
  Gain : Gain  Gain=Controller.KV *0.5
  Gain Scheduling : Subsystem
  Gain1 : Gain
  Rate Limiter : RateLimiter  RisingSlewLimit=2*pi/180  FallingSlewLimit=-2 * pi/180  SampleTimeMode=inherited
  Saturation : Saturate  UpperLimit=7.55*pi/30  LowerLimit=5*pi/30
  Saturation Dynamic : simulink/Discontinuities/Saturation Dynamic  OutMin=[]  OutMax=[]  OutDataTypeStr=Inherit: Same as second input  OutDataType=fixdt(1, 16)  OutScaling=2^-10  DoSatur=off
  Scope2 : Scope
  Sum1 : Sum  Inputs=|++
  Sum3 : Sum  Inputs=|+-
  Sum4 : Sum  Inputs=|+-
  BldPitch : Outport
  wires:
  Divide3/1 -> Sum4/2
  Sum3/1 -> Gain Scheduling/1(In1)
  Saturation Dynamic/1 -> Rate Limiter/1, Delay/1
  Compare To Constant/1 -> Divide3/1
  Constant/1 -> Sum4/1
  Constant1/1 -> Saturation Dynamic/1
  3/1 -> Compare To Constant/1, Divide3/2
  Delay/1 -> Gain Scheduling/3(In2)
  RotSpeed/1 -> Sum3/2
  Gain Scheduling/1(Out1) -> Sum1/1
  Sum1/1 -> Saturation Dynamic/2
  Gain/1 -> Sum1/2
  Nacelle Speed/1 -> Gain/1
  WindSpeed/1 -> 1-D Lookup Table/1  "Vhat"
  1-D Lookup Table/1 -> Gain1/1
  Gain1/1 -> Saturation Dynamic/3, Gain Scheduling/2(In3), Scope2/1
  Rate Limiter/1 -> BldPitch/1
  Sum4/1 -> Saturation/1
  Saturation/1 -> Sum3/1

== system LoFT_Example3/FOWT System/Subsystem13/FOWT3/Aerodynamics and Local Control Systems/Local Control Systems/Subsystem2 ==
  GenTorq : Inport
  BldPitch : Inport  Port=2
  Constant3 : Constant  Value=-Controller.torqueMax
  Gain 1 : Gain  Gain=Controller.SPS_kb/deg2rad(30)
  Gain 2 : Gain  Gain=Controller.omegaMax
  Gain 3 : Gain  Gain=-Controller.SPS_kt/Controller.torqueMax
  Sum5 : Sum  Inputs=|+-
  Sum6 : Sum  Inputs=|+-
  Delta_omega_g : Outport
  wires:
  Sum6/1 -> Gain 2/1
  Gain 1/1 -> Sum6/1
  Constant3/1 -> Sum5/2
  Gain 3/1 -> Sum6/2
  Sum5/1 -> Gain 3/1
  Gain 2/1 -> Delta_omega_g/1
  BldPitch/1 -> Gain 1/1
  GenTorq/1 -> Sum5/1

== system LoFT_Example3/FOWT System/Subsystem13/FOWT3/Aerodynamics and Local Control Systems/Local Control Systems/wind speed estimator ==
  In1 : Inport
  Discrete Filter : DiscreteFilter  Numerator=Controller.F.Wind.b  Denominator=Controller.F.Wind.a  InitialStates=2000
  Out1 : Outport
  wires:
  Discrete Filter/1 -> Out1/1
  In1/1 -> Discrete Filter/1

== system LoFT_Example3/FOWT System/Subsystem13/FOWT4/Aerodynamics and Local Control Systems/Local Control Systems/Subsystem ==
  WindSpeed : Inport
  2 : Inport  Port=2
  RotSpeed : Inport  Port=3
  Compare To Constant1 : simulink/Logic and Bit Operations/Compare To Constant  relop=>=  const=0  OutDataTypeStr=boolean
  Divide4 : Product  Inputs=**
  Gain5 : Gain  Gain=Controller.R.VS_KI
  Gain6 : Gain  Gain=Controller.R.VS_KP
  Integrator1 : Integrator  InitialCondition=Controller.torqueMax * 0.7  LimitOutput=on  UpperSaturationLimit=Controller.torqueMax
  Optimall TSR / Radius : Gain  Gain=Controller.R.VS_TSRopt/Controller.R.RotorRad
  Rate Limiter : RateLimiter  RisingSlewLimit=Controller.torqueMaxRate  FallingSlewLimit=-Controller.torqueMaxRate  SampleTimeMode=inherited
  Saturation : Saturate  UpperLimit=7.55*pi/30  LowerLimit=5*pi/30
  Saturation1 : Saturate  UpperLimit=Controller.torqueMax  LowerLimit=0
  Saturation2 : Saturate  UpperLimit=7.55*pi/30  LowerLimit=5*pi/30
  Scope2 : Scope
  Sum2 : Sum  Inputs=|+-
  Sum7 : Sum  Inputs=|+-
  Sum8 : Sum  Inputs=|++
  GenTorq : Outport
  wires:
  Gain6/1 -> Sum8/1
  WindSpeed/1 -> Optimall TSR / Radius/1
  Sum7/1 -> Saturation/1
  Divide4/1 -> Scope2/1, Sum7/2
  2/1 -> Compare To Constant1/1, Divide4/2
  Rate Limiter/1 -> GenTorq/1
  Saturation/1 -> Sum2/1
  Compare To Constant1/1 -> Divide4/1
  Sum2/1 -> Gain6/1, Gain5/1
  Integrator1/1 -> Sum8/2
  Gain5/1 -> Integrator1/1
  Sum8/1 -> Saturation1/1
  RotSpeed/1 -> Sum2/2
  Saturation1/1 -> Rate Limiter/1
  Saturation2/1 -> Sum7/1
  Optimall TSR / Radius/1 -> Saturation2/1

== system LoFT_Example3/FOWT System/Subsystem13/FOWT4/Aerodynamics and Local Control Systems/Local Control Systems/Subsystem1 ==
  RotSpeed : Inport
  WindSpeed : Inport  Port=2
  3 : Inport  Port=3
  Nacelle Speed : Inport  Port=4
  1-D Lookup Table : Lookup_n-D  NumberOfTableDimensions=1  BreakpointsForDimension1=Controller.R.PS_WindSpeeds  Table=Controller.R.PS_BldPitchMin  InternalRulePriority=Speed  RndMeth=Simplest
  Compare To Constant : simulink/Logic and Bit Operations/Compare To Constant  relop=<=  const=0  OutDataTypeStr=boolean
  Constant : Constant  Value=7.55*pi/30
  Constant1 : Constant  Value=90*pi/180
  Delay : Delay  DelayLength=1  InitialCondition=0
  Divide3 : Product  Inputs=**
  Gain : Gain  Gain=Controller.KV *0.5
  Gain Scheduling : Subsystem
  Gain1 : Gain
  Rate Limiter : RateLimiter  RisingSlewLimit=2*pi/180  FallingSlewLimit=-2 * pi/180  SampleTimeMode=inherited
  Saturation : Saturate  UpperLimit=7.55*pi/30  LowerLimit=5*pi/30
  Saturation Dynamic : simulink/Discontinuities/Saturation Dynamic  OutMin=[]  OutMax=[]  OutDataTypeStr=Inherit: Same as second input  OutDataType=fixdt(1, 16)  OutScaling=2^-10  DoSatur=off
  Scope2 : Scope
  Sum1 : Sum  Inputs=|++
  Sum3 : Sum  Inputs=|+-
  Sum4 : Sum  Inputs=|+-
  BldPitch : Outport
  wires:
  Saturation/1 -> Sum3/1
  Sum4/1 -> Saturation/1
  Rate Limiter/1 -> BldPitch/1
  Gain1/1 -> Scope2/1, Gain Scheduling/2(In3), Saturation Dynamic/3
  1-D Lookup Table/1 -> Gain1/1
  WindSpeed/1 -> 1-D Lookup Table/1  "Vhat"
  Nacelle Speed/1 -> Gain/1
  Gain/1 -> Sum1/2
  Sum1/1 -> Saturation Dynamic/2
  Gain Scheduling/1(Out1) -> Sum1/1
  RotSpeed/1 -> Sum3/2
  Delay/1 -> Gain Scheduling/3(In2)
  3/1 -> Divide3/2, Compare To Constant/1
  Constant1/1 -> Saturation Dynamic/1
  Constant/1 -> Sum4/1
  Compare To Constant/1 -> Divide3/1
  Saturation Dynamic/1 -> Delay/1, Rate Limiter/1
  Sum3/1 -> Gain Scheduling/1(In1)
  Divide3/1 -> Sum4/2

== system LoFT_Example3/FOWT System/Subsystem13/FOWT4/Aerodynamics and Local Control Systems/Local Control Systems/Subsystem2 ==
  GenTorq : Inport
  BldPitch : Inport  Port=2
  Constant3 : Constant  Value=-Controller.torqueMax
  Gain 1 : Gain  Gain=Controller.SPS_kb/deg2rad(30)
  Gain 2 : Gain  Gain=Controller.omegaMax
  Gain 3 : Gain  Gain=-Controller.SPS_kt/Controller.torqueMax
  Sum5 : Sum  Inputs=|+-
  Sum6 : Sum  Inputs=|+-
  Delta_omega_g : Outport
  wires:
  GenTorq/1 -> Sum5/1
  BldPitch/1 -> Gain 1/1
  Gain 2/1 -> Delta_omega_g/1
  Sum5/1 -> Gain 3/1
  Gain 3/1 -> Sum6/2
  Constant3/1 -> Sum5/2
  Gain 1/1 -> Sum6/1
  Sum6/1 -> Gain 2/1

== system LoFT_Example3/FOWT System/Subsystem13/FOWT4/Aerodynamics and Local Control Systems/Local Control Systems/wind speed estimator ==
  In1 : Inport
  Discrete Filter : DiscreteFilter  Numerator=Controller.F.Wind.b  Denominator=Controller.F.Wind.a  InitialStates=2000
  Out1 : Outport
  wires:
  In1/1 -> Discrete Filter/1
  Discrete Filter/1 -> Out1/1

== system LoFT_Example3/FOWT System/Subsystem13/FOWT5/Aerodynamics and Local Control Systems/Local Control Systems/Subsystem ==
  WindSpeed : Inport
  2 : Inport  Port=2
  RotSpeed : Inport  Port=3
  Compare To Constant1 : simulink/Logic and Bit Operations/Compare To Constant  relop=>=  const=0  OutDataTypeStr=boolean
  Divide4 : Product  Inputs=**
  Gain5 : Gain  Gain=Controller.R.VS_KI
  Gain6 : Gain  Gain=Controller.R.VS_KP
  Integrator1 : Integrator  InitialCondition=Controller.torqueMax * 0.7  LimitOutput=on  UpperSaturationLimit=Controller.torqueMax
  Optimall TSR / Radius : Gain  Gain=Controller.R.VS_TSRopt/Controller.R.RotorRad
  Rate Limiter : RateLimiter  RisingSlewLimit=Controller.torqueMaxRate  FallingSlewLimit=-Controller.torqueMaxRate  SampleTimeMode=inherited
  Saturation : Saturate  UpperLimit=7.55*pi/30  LowerLimit=5*pi/30
  Saturation1 : Saturate  UpperLimit=Controller.torqueMax  LowerLimit=0
  Saturation2 : Saturate  UpperLimit=7.55*pi/30  LowerLimit=5*pi/30
  Scope2 : Scope
  Sum2 : Sum  Inputs=|+-
  Sum7 : Sum  Inputs=|+-
  Sum8 : Sum  Inputs=|++
  GenTorq : Outport
  wires:
  Optimall TSR / Radius/1 -> Saturation2/1
  Saturation2/1 -> Sum7/1
  Saturation1/1 -> Rate Limiter/1
  RotSpeed/1 -> Sum2/2
  Sum8/1 -> Saturation1/1
  Gain5/1 -> Integrator1/1
  Integrator1/1 -> Sum8/2
  Sum2/1 -> Gain5/1, Gain6/1
  Compare To Constant1/1 -> Divide4/1
  Saturation/1 -> Sum2/1
  Rate Limiter/1 -> GenTorq/1
  2/1 -> Divide4/2, Compare To Constant1/1
  Divide4/1 -> Sum7/2, Scope2/1
  Sum7/1 -> Saturation/1
  WindSpeed/1 -> Optimall TSR / Radius/1
  Gain6/1 -> Sum8/1

== system LoFT_Example3/FOWT System/Subsystem13/FOWT5/Aerodynamics and Local Control Systems/Local Control Systems/Subsystem1 ==
  RotSpeed : Inport
  WindSpeed : Inport  Port=2
  3 : Inport  Port=3
  Nacelle Speed : Inport  Port=4
  1-D Lookup Table : Lookup_n-D  NumberOfTableDimensions=1  BreakpointsForDimension1=Controller.R.PS_WindSpeeds  Table=Controller.R.PS_BldPitchMin  InternalRulePriority=Speed  RndMeth=Simplest
  Compare To Constant : simulink/Logic and Bit Operations/Compare To Constant  relop=<=  const=0  OutDataTypeStr=boolean
  Constant : Constant  Value=7.55*pi/30
  Constant1 : Constant  Value=90*pi/180
  Delay : Delay  DelayLength=1  InitialCondition=0
  Divide3 : Product  Inputs=**
  Gain : Gain  Gain=Controller.KV *0.5
  Gain Scheduling : Subsystem
  Gain1 : Gain
  Rate Limiter : RateLimiter  RisingSlewLimit=2*pi/180  FallingSlewLimit=-2 * pi/180  SampleTimeMode=inherited
  Saturation : Saturate  UpperLimit=7.55*pi/30  LowerLimit=5*pi/30
  Saturation Dynamic : simulink/Discontinuities/Saturation Dynamic  OutMin=[]  OutMax=[]  OutDataTypeStr=Inherit: Same as second input  OutDataType=fixdt(1, 16)  OutScaling=2^-10  DoSatur=off
  Scope2 : Scope
  Sum1 : Sum  Inputs=|++
  Sum3 : Sum  Inputs=|+-
  Sum4 : Sum  Inputs=|+-
  BldPitch : Outport
  wires:
  Divide3/1 -> Sum4/2
  Sum3/1 -> Gain Scheduling/1(In1)
  Saturation Dynamic/1 -> Rate Limiter/1, Delay/1
  Compare To Constant/1 -> Divide3/1
  Constant/1 -> Sum4/1
  Constant1/1 -> Saturation Dynamic/1
  3/1 -> Compare To Constant/1, Divide3/2
  Delay/1 -> Gain Scheduling/3(In2)
  RotSpeed/1 -> Sum3/2
  Gain Scheduling/1(Out1) -> Sum1/1
  Sum1/1 -> Saturation Dynamic/2
  Gain/1 -> Sum1/2
  Nacelle Speed/1 -> Gain/1
  WindSpeed/1 -> 1-D Lookup Table/1  "Vhat"
  1-D Lookup Table/1 -> Gain1/1
  Gain1/1 -> Saturation Dynamic/3, Gain Scheduling/2(In3), Scope2/1
  Rate Limiter/1 -> BldPitch/1
  Sum4/1 -> Saturation/1
  Saturation/1 -> Sum3/1

== system LoFT_Example3/FOWT System/Subsystem13/FOWT5/Aerodynamics and Local Control Systems/Local Control Systems/Subsystem2 ==
  GenTorq : Inport
  BldPitch : Inport  Port=2
  Constant3 : Constant  Value=-Controller.torqueMax
  Gain 1 : Gain  Gain=Controller.SPS_kb/deg2rad(30)
  Gain 2 : Gain  Gain=Controller.omegaMax
  Gain 3 : Gain  Gain=-Controller.SPS_kt/Controller.torqueMax
  Sum5 : Sum  Inputs=|+-
  Sum6 : Sum  Inputs=|+-
  Delta_omega_g : Outport
  wires:
  Sum6/1 -> Gain 2/1
  Gain 1/1 -> Sum6/1
  Constant3/1 -> Sum5/2
  Gain 3/1 -> Sum6/2
  Sum5/1 -> Gain 3/1
  Gain 2/1 -> Delta_omega_g/1
  BldPitch/1 -> Gain 1/1
  GenTorq/1 -> Sum5/1

== system LoFT_Example3/FOWT System/Subsystem13/FOWT5/Aerodynamics and Local Control Systems/Local Control Systems/wind speed estimator ==
  In1 : Inport
  Discrete Filter : DiscreteFilter  Numerator=Controller.F.Wind.b  Denominator=Controller.F.Wind.a  InitialStates=2000
  Out1 : Outport
  wires:
  Discrete Filter/1 -> Out1/1
  In1/1 -> Discrete Filter/1

== system LoFT_Example3/FOWT System/Subsystem13/FOWT6/Aerodynamics and Local Control Systems/Local Control Systems/Subsystem ==
  WindSpeed : Inport
  2 : Inport  Port=2
  RotSpeed : Inport  Port=3
  Compare To Constant1 : simulink/Logic and Bit Operations/Compare To Constant  relop=>=  const=0  OutDataTypeStr=boolean
  Divide4 : Product  Inputs=**
  Gain5 : Gain  Gain=Controller.R.VS_KI
  Gain6 : Gain  Gain=Controller.R.VS_KP
  Integrator1 : Integrator  InitialCondition=Controller.torqueMax * 0.7  LimitOutput=on  UpperSaturationLimit=Controller.torqueMax
  Optimall TSR / Radius : Gain  Gain=Controller.R.VS_TSRopt/Controller.R.RotorRad
  Rate Limiter : RateLimiter  RisingSlewLimit=Controller.torqueMaxRate  FallingSlewLimit=-Controller.torqueMaxRate  SampleTimeMode=inherited
  Saturation : Saturate  UpperLimit=7.55*pi/30  LowerLimit=5*pi/30
  Saturation1 : Saturate  UpperLimit=Controller.torqueMax  LowerLimit=0
  Saturation2 : Saturate  UpperLimit=7.55*pi/30  LowerLimit=5*pi/30
  Scope2 : Scope
  Sum2 : Sum  Inputs=|+-
  Sum7 : Sum  Inputs=|+-
  Sum8 : Sum  Inputs=|++
  GenTorq : Outport
  wires:
  Gain6/1 -> Sum8/1
  WindSpeed/1 -> Optimall TSR / Radius/1
  Sum7/1 -> Saturation/1
  Divide4/1 -> Scope2/1, Sum7/2
  2/1 -> Compare To Constant1/1, Divide4/2
  Rate Limiter/1 -> GenTorq/1
  Saturation/1 -> Sum2/1
  Compare To Constant1/1 -> Divide4/1
  Sum2/1 -> Gain6/1, Gain5/1
  Integrator1/1 -> Sum8/2
  Gain5/1 -> Integrator1/1
  Sum8/1 -> Saturation1/1
  RotSpeed/1 -> Sum2/2
  Saturation1/1 -> Rate Limiter/1
  Saturation2/1 -> Sum7/1
  Optimall TSR / Radius/1 -> Saturation2/1

== system LoFT_Example3/FOWT System/Subsystem13/FOWT6/Aerodynamics and Local Control Systems/Local Control Systems/Subsystem1 ==
  RotSpeed : Inport
  WindSpeed : Inport  Port=2
  3 : Inport  Port=3
  Nacelle Speed : Inport  Port=4
  1-D Lookup Table : Lookup_n-D  NumberOfTableDimensions=1  BreakpointsForDimension1=Controller.R.PS_WindSpeeds  Table=Controller.R.PS_BldPitchMin  InternalRulePriority=Speed  RndMeth=Simplest
  Compare To Constant : simulink/Logic and Bit Operations/Compare To Constant  relop=<=  const=0  OutDataTypeStr=boolean
  Constant : Constant  Value=7.55*pi/30
  Constant1 : Constant  Value=90*pi/180
  Delay : Delay  DelayLength=1  InitialCondition=0
  Divide3 : Product  Inputs=**
  Gain : Gain  Gain=Controller.KV *0.5
  Gain Scheduling : Subsystem
  Gain1 : Gain
  Rate Limiter : RateLimiter  RisingSlewLimit=2*pi/180  FallingSlewLimit=-2 * pi/180  SampleTimeMode=inherited
  Saturation : Saturate  UpperLimit=7.55*pi/30  LowerLimit=5*pi/30
  Saturation Dynamic : simulink/Discontinuities/Saturation Dynamic  OutMin=[]  OutMax=[]  OutDataTypeStr=Inherit: Same as second input  OutDataType=fixdt(1, 16)  OutScaling=2^-10  DoSatur=off
  Scope2 : Scope
  Sum1 : Sum  Inputs=|++
  Sum3 : Sum  Inputs=|+-
  Sum4 : Sum  Inputs=|+-
  BldPitch : Outport
  wires:
  Saturation/1 -> Sum3/1
  Sum4/1 -> Saturation/1
  Rate Limiter/1 -> BldPitch/1
  Gain1/1 -> Scope2/1, Gain Scheduling/2(In3), Saturation Dynamic/3
  1-D Lookup Table/1 -> Gain1/1
  WindSpeed/1 -> 1-D Lookup Table/1  "Vhat"
  Nacelle Speed/1 -> Gain/1
  Gain/1 -> Sum1/2
  Sum1/1 -> Saturation Dynamic/2
  Gain Scheduling/1(Out1) -> Sum1/1
  RotSpeed/1 -> Sum3/2
  Delay/1 -> Gain Scheduling/3(In2)
  3/1 -> Divide3/2, Compare To Constant/1
  Constant1/1 -> Saturation Dynamic/1
  Constant/1 -> Sum4/1
  Compare To Constant/1 -> Divide3/1
  Saturation Dynamic/1 -> Delay/1, Rate Limiter/1
  Sum3/1 -> Gain Scheduling/1(In1)
  Divide3/1 -> Sum4/2

== system LoFT_Example3/FOWT System/Subsystem13/FOWT6/Aerodynamics and Local Control Systems/Local Control Systems/Subsystem2 ==
  GenTorq : Inport
  BldPitch : Inport  Port=2
  Constant3 : Constant  Value=-Controller.torqueMax
  Gain 1 : Gain  Gain=Controller.SPS_kb/deg2rad(30)
  Gain 2 : Gain  Gain=Controller.omegaMax
  Gain 3 : Gain  Gain=-Controller.SPS_kt/Controller.torqueMax
  Sum5 : Sum  Inputs=|+-
  Sum6 : Sum  Inputs=|+-
  Delta_omega_g : Outport
  wires:
  GenTorq/1 -> Sum5/1
  BldPitch/1 -> Gain 1/1
  Gain 2/1 -> Delta_omega_g/1
  Sum5/1 -> Gain 3/1
  Gain 3/1 -> Sum6/2
  Constant3/1 -> Sum5/2
  Gain 1/1 -> Sum6/1
  Sum6/1 -> Gain 2/1

== system LoFT_Example3/FOWT System/Subsystem13/FOWT6/Aerodynamics and Local Control Systems/Local Control Systems/wind speed estimator ==
  In1 : Inport
  Discrete Filter : DiscreteFilter  Numerator=Controller.F.Wind.b  Denominator=Controller.F.Wind.a  InitialStates=2000
  Out1 : Outport
  wires:
  In1/1 -> Discrete Filter/1
  Discrete Filter/1 -> Out1/1
